simulink model "saturateur"  (R2020a)
settings: Solver=VariableStepAuto  StartTime=0.0  StopTime=10.0  RelTol=1e-3
undefined symbols (not defined in the file): K, Kfiltre, S, Tc3, Tc4, Tg, Tr1, Tr2, Ubatt
settings Model: Creator=housni  LastModifiedBy=housni

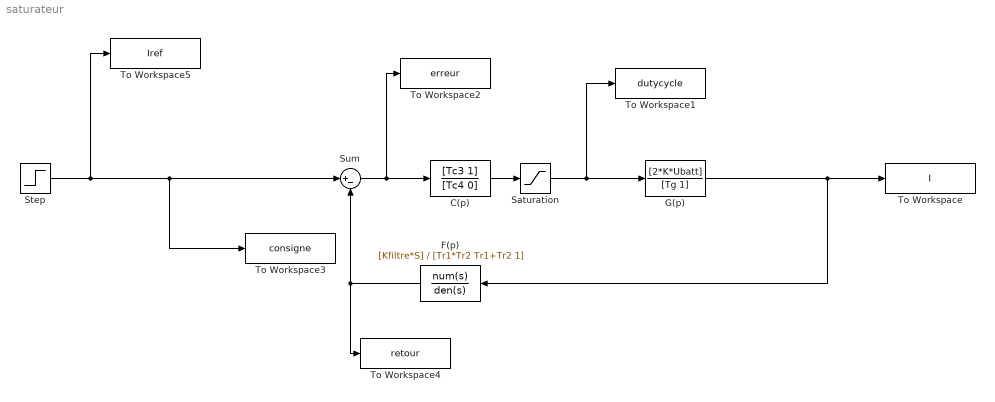
== system saturateur ==
  C(p) : TransferFcn  Numerator=[Tc3 1]  Denominator=[Tc4 0]
  F(p) : TransferFcn  Numerator=[Kfiltre*S]  Denominator=[Tr1*Tr2 Tr1+Tr2 1]
  G(p) : TransferFcn  Numerator=[2*K*Ubatt]  Denominator=[Tg 1]
  Saturation : Saturate
  Step : Step  After=1.65  SampleTime=0
  Sum : Sum  Inputs=|+-
  To Workspace : ToWorkspace  VariableName=I  SaveFormat=Timeseries  SampleTime=-1
  To Workspace1 : ToWorkspace  VariableName=dutycycle  SaveFormat=Timeseries  SampleTime=-1
  To Workspace2 : ToWorkspace  VariableName=erreur  SaveFormat=Timeseries  SampleTime=-1
  To Workspace3 : ToWorkspace  VariableName=consigne  SaveFormat=Timeseries  SampleTime=-1
  To Workspace4 : ToWorkspace  VariableName=retour  SaveFormat=Timeseries  SampleTime=-1
  To Workspace5 : ToWorkspace  VariableName=Iref  SaveFormat=Timeseries  SampleTime=-1
  wires:
  F(p)/1 -> To Workspace4/1, Sum/2
  Sum/1 -> To Workspace2/1, C(p)/1
  G(p)/1 -> F(p)/1, To Workspace/1
  Step/1 -> To Workspace3/1, Sum/1, To Workspace5/1
  C(p)/1 -> Saturation/1
  Saturation/1 -> To Workspace1/1, G(p)/1
